simulink model "slip_ratio_only"  (R2020b)
settings: Solver=VariableStepAuto  StartTime=0.0  StopTime=10.0  RelTol=1e-3
undefined symbols (not defined in the file): jw, m, r
settings Model: Creator=K E S SRINIVAS  LastModifiedBy=K E S SRINIVAS

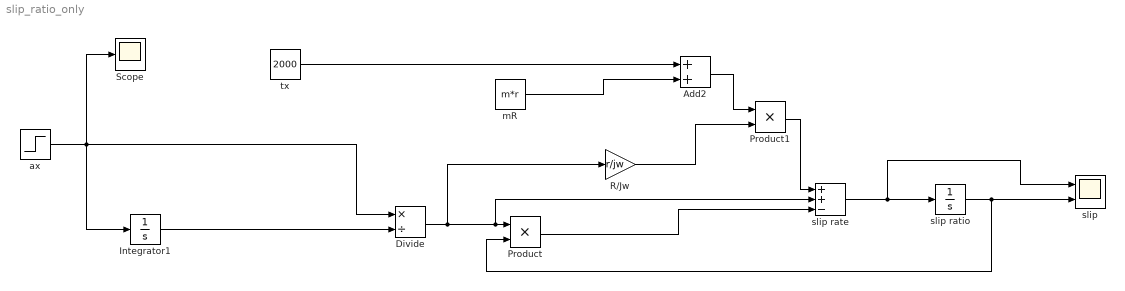
== system slip_ratio_only ==
  Add2 : Sum
  Divide : Product  Inputs=*/
  Integrator1 : Integrator
  Product : Product
  Product1 : Product
  R/Jw : Gain  Gain=r/jw
  Scope : Scope
  ax : Step  After=20  SampleTime=0
  mR : Constant  Value=m*r
  slip : Scope  NumInputPorts=2
  slip rate : Sum  Inputs=++-
  slip ratio : Integrator
  tx : Constant  Value=2000
  wires:
  slip ratio/1 -> slip/2, Product/2
  R/Jw/1 -> Product1/2
  Integrator1/1 -> Divide/2
  tx/1 -> Add2/1
  Divide/1 -> R/Jw/1, slip rate/2, Product/1
  Add2/1 -> Product1/1
  mR/1 -> Add2/2
  slip rate/1 -> slip/1, slip ratio/1
  Product/1 -> slip rate/3
  Product1/1 -> slip rate/1
  ax/1 -> Scope/1, Divide/1, Integrator1/1
